simulink model "Example_Subsystem0_2016b"  (Simulink 8.8)
settings: Solver=FixedStepDiscrete  StartTime=0.0  StopTime=10.0  FixedStep=0.0003125  RelTol=1e-3  EnableMultiTasking=on
settings Model: Creator=monika  LastModifiedBy=monika
settings OptimizationCC: ExpressionDepthLimit=2147483647  LifeSpan=1
settings DebuggingCC: CheckSSInitialOutputMsg=off  SolverPrmCheckMsg=warning
settings RTWCC: SystemTargetFile=ert.tlc  TemplateMakefile=ert_default_tmf  Description=Embedded Coder
settings CodeAppCC: IgnoreCustomStorageClasses=off  CustomSymbolStrType=$N$R$M  InternalIdentifier=Classic
settings ERTTargetCC: MultiwordLength=2048  GenerateSampleERTMain=on  ERTCustomFileTemplate=example_file_process.tlc  ConvertIfToSwitch=off  SuppressUnreachableDefaultCases=off

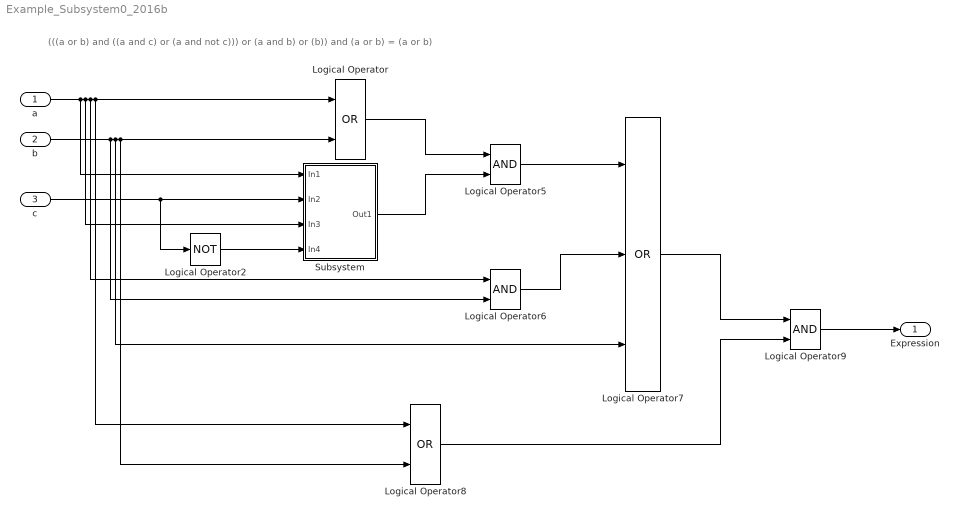
== system Example_Subsystem0_2016b ==
  note: (((a or b) and ((a and c) or (a and not c))) or (a and b) or (b)) and (a or b) = (a or b)
  a : Inport
  b : Inport  Port=2
  c : Inport  Port=3
  Logical Operator : Logic  Operator=OR  AllPortsSameDT=off  OutDataTypeStr=boolean
  Logical Operator2 : Logic  Operator=NOT  AllPortsSameDT=off  OutDataTypeStr=boolean
  Logical Operator5 : Logic  AllPortsSameDT=off  OutDataTypeStr=boolean
  Logical Operator6 : Logic  AllPortsSameDT=off  OutDataTypeStr=boolean
  Logical Operator7 : Logic  Operator=OR  Inputs=3  AllPortsSameDT=off  OutDataTypeStr=boolean
  Logical Operator8 : Logic  Operator=OR  AllPortsSameDT=off  OutDataTypeStr=boolean
  Logical Operator9 : Logic  AllPortsSameDT=off  OutDataTypeStr=boolean
  Subsystem : Subsystem
  Expression : Outport
  wires:
  Logical Operator2/1 -> Subsystem/4(In4)
  Logical Operator/1 -> Logical Operator5/1
  Subsystem/1(Out1) -> Logical Operator5/2
  Logical Operator5/1 -> Logical Operator7/1
  Logical Operator6/1 -> Logical Operator7/2
  c/1 -> Subsystem/2(In2), Logical Operator2/1
  Logical Operator9/1 -> Expression/1
  Logical Operator7/1 -> Logical Operator9/1
  Logical Operator8/1 -> Logical Operator9/2
  a/1 -> Subsystem/1(In1), Subsystem/3(In3), Logical Operator6/1, Logical Operator/1, Logical Operator8/1
  b/1 -> Logical Operator6/2, Logical Operator7/3, Logical Operator/2, Logical Operator8/2

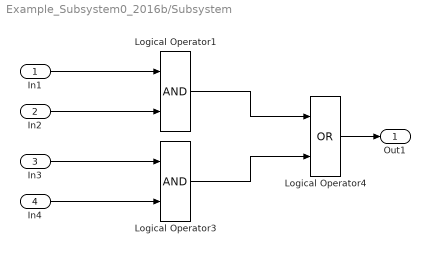
== system Example_Subsystem0_2016b/Subsystem ==
  In1 : Inport
  In2 : Inport  Port=2
  In3 : Inport  Port=3
  In4 : Inport  Port=4
  Logical Operator1 : Logic  AllPortsSameDT=off  OutDataTypeStr=boolean
  Logical Operator3 : Logic  AllPortsSameDT=off  OutDataTypeStr=boolean
  Logical Operator4 : Logic  Operator=OR  AllPortsSameDT=off  OutDataTypeStr=boolean
  Out1 : Outport
  wires:
  Logical Operator4/1 -> Out1/1
  In1/1 -> Logical Operator1/1
  In2/1 -> Logical Operator1/2
  Logical Operator1/1 -> Logical Operator4/1
  Logical Operator3/1 -> Logical Operator4/2
  In3/1 -> Logical Operator3/1
  In4/1 -> Logical Operator3/2
